simulink model "Ejerciciocasa"  (R2013a)
settings: Solver=ode45  StartTime=0.0  StopTime=10.0  RelTol=1e-3
settings Model: Creator=CONTROL PLC 001  LastModifiedBy=CONTROL PLC 001

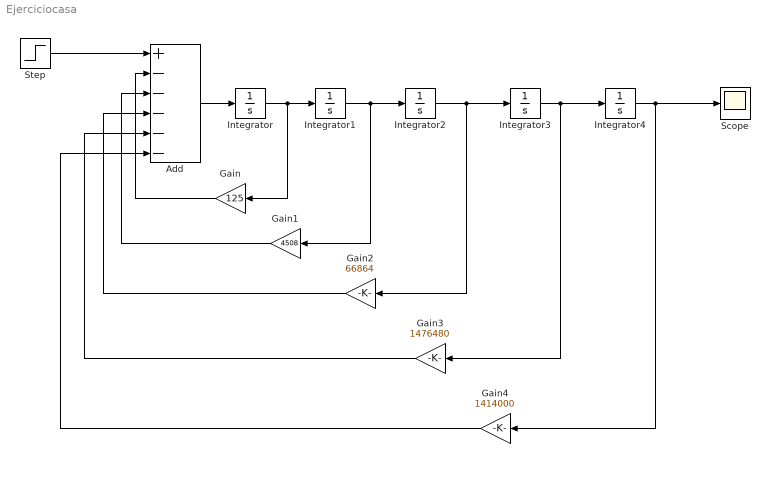
== system Ejerciciocasa ==
  Add : Sum  RequirementInfo="{}  %GIDa_dbeb203a_0255_405a_ba3d_83ec77c7e772"  Inputs=+-----
  Gain : Gain  Gain=125
  Gain1 : Gain  Gain=4508
  Gain2 : Gain  Gain=66864
  Gain3 : Gain  Gain=1476480
  Gain4 : Gain  Gain=1414000
  Integrator{,1..4} (5 alike) : Integrator
  Scope : Scope
  Step : Step  SampleTime=0
  wires:
  Add/1 -> Integrator/1
  Integrator/1 -> Gain/1, Integrator1/1
  Integrator1/1 -> Gain1/1, Integrator2/1
  Integrator2/1 -> Gain2/1, Integrator3/1
  Gain/1 -> Add/2
  Gain1/1 -> Add/3
  Gain2/1 -> Add/4
  Integrator3/1 -> Integrator4/1, Gain3/1
  Gain3/1 -> Add/5
  Integrator4/1 -> Gain4/1, Scope/1
  Gain4/1 -> Add/6
  Step/1 -> Add/1
